simulink model "snap2_f_200msps_64i_4096c"  (R2019a)
settings: Solver=VariableStepDiscrete  StartTime=0.0  StopTime=10.0  RelTol=1e-3
undefined symbols (not defined in the file or in its folder): datetime, posixtime
libraries: xbsIndex_r4 x21354, casper_library_misc x297, casper_library_delays x19, xps_library x14, casper_library_sources x4
(part 17 of 217)

== system snap2_f_200msps_64i_4096c/cosmic_ray/count_thresh_exceeded2 ==
  pps_in : Inport
  din : Inport  Port=2
  AddSub : xbsIndex_r4/AddSub  mode=Subtraction  use_carryin=off  use_carryout=off  en=off  latency=1  precision=User Defined  arith_type=Unsigned  n_bits=5  bin_pt=0  quantization=Truncate  overflow=Wrap  use_behavioral_HDL=on  hw_selection=Fabric  pipelined=off  dbl_ovrd=off  block_type=addsub
  AddSub1 : xbsIndex_r4/AddSub  mode=Subtraction  use_carryin=off  use_carryout=off  en=off  latency=1  precision=User Defined  arith_type=Unsigned  n_bits=5  bin_pt=0  quantization=Truncate  overflow=Wrap  use_behavioral_HDL=on  hw_selection=Fabric  pipelined=off  dbl_ovrd=off  block_type=addsub
  Constant : xbsIndex_r4/Constant  const=32  gui_display_data_type=Fixed-point  arith_type=Unsigned  n_bits=6  bin_pt=0  preci_type=Single  exp_width=8  frac_width=24  explicit_period=off  period=1  equ=P=C  opselect=C  inp2=PCIN>>17  opr=+  inp1=P  carry=CIN  dbl_ovrd=off  block_type=constant
  Constant1 : xbsIndex_r4/Constant  const=1.0  gui_display_data_type=Fixed-point  arith_type=Unsigned  n_bits=1  bin_pt=0  preci_type=Single  exp_width=8  frac_width=24  explicit_period=off  period=1  equ=P=C  opselect=C  inp2=PCIN>>17  opr=+  inp1=P  carry=CIN  dbl_ovrd=off  block_type=constant
  Constant2 : xbsIndex_r4/Constant  const=1.0  gui_display_data_type=Fixed-point  arith_type=Unsigned  n_bits=1  bin_pt=0  preci_type=Single  exp_width=8  frac_width=24  explicit_period=off  period=1  equ=P=C  opselect=C  inp2=PCIN>>17  opr=+  inp1=P  carry=CIN  dbl_ovrd=off  block_type=constant
  Convert : xbsIndex_r4/Convert  gui_display_data_type=Boolean  arith_type=Boolean  n_bits=16  bin_pt=14  float_type=Single  exp_bits=8  fraction_bits=24  quantization=Truncate  overflow=Wrap  en=off  latency=1  pipeline=off  dbl_ovrd=off  block_type=convert
  Counter{2,6..68} (64 alike) : xbsIndex_r4/Counter  cnt_type=Count Limited  cnt_to=Inf  operation=Up  start_count=0  cnt_by_val=1  arith_type=Unsigned  n_bits=32  bin_pt=0  load_pin=off  rst=on  en=on  explicit_period=on  period=1  use_behavioral_HDL=off  implementation=Fabric  dbl_ovrd=off  block_type=counter
  Counter69 : xbsIndex_r4/Counter  cnt_type=Free Running  cnt_to=Inf  operation=Up  start_count=0  cnt_by_val=1  arith_type=Unsigned  n_bits=5  bin_pt=0  load_pin=off  rst=on  en=on  explicit_period=on  period=1  use_behavioral_HDL=off  implementation=Fabric  dbl_ovrd=off  block_type=counter
  Delay1 : xbsIndex_r4/Delay  rst=off  infoeditControl=Selection of Reset will increase slice count due to use of real FFs and instead of SRLs  en=off  latency=5  reg_retiming=on  dbl_ovrd=off  block_type=delay
  Delay10 : xbsIndex_r4/Delay  rst=off  infoeditControl=Selection of Reset will increase slice count due to use of real FFs and instead of SRLs  en=off  latency=13  reg_retiming=on  dbl_ovrd=off  block_type=delay
  Delay100 : xbsIndex_r4/Delay  rst=off  infoeditControl=Selection of Reset will increase slice count due to use of real FFs and instead of SRLs  en=off  latency=2  reg_retiming=on  dbl_ovrd=off  block_type=delay
  Delay101 : xbsIndex_r4/Delay  rst=off  infoeditControl=Selection of Reset will increase slice count due to use of real FFs and instead of SRLs  en=off  latency=3  reg_retiming=on  dbl_ovrd=off  block_type=delay
  Delay102 : xbsIndex_r4/Delay  rst=off  infoeditControl=Selection of Reset will increase slice count due to use of real FFs and instead of SRLs  en=off  latency=4  reg_retiming=on  dbl_ovrd=off  block_type=delay
  Delay11 : xbsIndex_r4/Delay  rst=off  infoeditControl=Selection of Reset will increase slice count due to use of real FFs and instead of SRLs  en=off  latency=14  reg_retiming=on  dbl_ovrd=off  block_type=delay
  Delay12 : xbsIndex_r4/Delay  rst=off  infoeditControl=Selection of Reset will increase slice count due to use of real FFs and instead of SRLs  en=off  latency=15  reg_retiming=on  dbl_ovrd=off  block_type=delay
  Delay13 : xbsIndex_r4/Delay  rst=off  infoeditControl=Selection of Reset will increase slice count due to use of real FFs and instead of SRLs  en=off  latency=16  reg_retiming=on  dbl_ovrd=off  block_type=delay
  Delay14 : xbsIndex_r4/Delay  rst=off  infoeditControl=Selection of Reset will increase slice count due to use of real FFs and instead of SRLs  en=off  latency=9  reg_retiming=on  dbl_ovrd=off  block_type=delay
  Delay15 : xbsIndex_r4/Delay  rst=off  infoeditControl=Selection of Reset will increase slice count due to use of real FFs and instead of SRLs  en=off  latency=10  reg_retiming=on  dbl_ovrd=off  block_type=delay
  Delay16 : xbsIndex_r4/Delay  rst=off  infoeditControl=Selection of Reset will increase slice count due to use of real FFs and instead of SRLs  en=off  latency=11  reg_retiming=on  dbl_ovrd=off  block_type=delay
  Delay17 : xbsIndex_r4/Delay  rst=off  infoeditControl=Selection of Reset will increase slice count due to use of real FFs and instead of SRLs  en=off  latency=12  reg_retiming=on  dbl_ovrd=off  block_type=delay
  Delay18 : xbsIndex_r4/Delay  rst=off  infoeditControl=Selection of Reset will increase slice count due to use of real FFs and instead of SRLs  en=off  latency=21  reg_retiming=on  dbl_ovrd=off  block_type=delay
  Delay19 : xbsIndex_r4/Delay  rst=off  infoeditControl=Selection of Reset will increase slice count due to use of real FFs and instead of SRLs  en=off  latency=22  reg_retiming=on  dbl_ovrd=off  block_type=delay
  Delay2 : xbsIndex_r4/Delay  rst=off  infoeditControl=Selection of Reset will increase slice count due to use of real FFs and instead of SRLs  en=off  latency=6  reg_retiming=on  dbl_ovrd=off  block_type=delay
  Delay20 : xbsIndex_r4/Delay  rst=off  infoeditControl=Selection of Reset will increase slice count due to use of real FFs and instead of SRLs  en=off  latency=23  reg_retiming=on  dbl_ovrd=off  block_type=delay
  Delay21 : xbsIndex_r4/Delay  rst=off  infoeditControl=Selection of Reset will increase slice count due to use of real FFs and instead of SRLs  en=off  latency=24  reg_retiming=on  dbl_ovrd=off  block_type=delay
  Delay22 : xbsIndex_r4/Delay  rst=off  infoeditControl=Selection of Reset will increase slice count due to use of real FFs and instead of SRLs  en=off  latency=29  reg_retiming=on  dbl_ovrd=off  block_type=delay
  Delay23 : xbsIndex_r4/Delay  rst=off  infoeditControl=Selection of Reset will increase slice count due to use of real FFs and instead of SRLs  en=off  latency=30  reg_retiming=on  dbl_ovrd=off  block_type=delay
  Delay24 : xbsIndex_r4/Delay  rst=off  infoeditControl=Selection of Reset will increase slice count due to use of real FFs and instead of SRLs  en=off  latency=31  reg_retiming=on  dbl_ovrd=off  block_type=delay
  Delay{25,34,38..40,70,99} (7 alike) : xbsIndex_r4/Delay  rst=off  infoeditControl=Selection of Reset will increase slice count due to use of real FFs and instead of SRLs  en=off  latency=1  reg_retiming=on  dbl_ovrd=off  block_type=delay
  Delay26 : xbsIndex_r4/Delay  rst=off  infoeditControl=Selection of Reset will increase slice count due to use of real FFs and instead of SRLs  en=off  latency=25  reg_retiming=on  dbl_ovrd=off  block_type=delay
  Delay27 : xbsIndex_r4/Delay  rst=off  infoeditControl=Selection of Reset will increase slice count due to use of real FFs and instead of SRLs  en=off  latency=26  reg_retiming=on  dbl_ovrd=off  block_type=delay
  Delay28 : xbsIndex_r4/Delay  rst=off  infoeditControl=Selection of Reset will increase slice count due to use of real FFs and instead of SRLs  en=off  latency=27  reg_retiming=on  dbl_ovrd=off  block_type=delay
  Delay29 : xbsIndex_r4/Delay  rst=off  infoeditControl=Selection of Reset will increase slice count due to use of real FFs and instead of SRLs  en=off  latency=28  reg_retiming=on  dbl_ovrd=off  block_type=delay
  Delay3 : xbsIndex_r4/Delay  rst=off  infoeditControl=Selection of Reset will increase slice count due to use of real FFs and instead of SRLs  en=off  latency=7  reg_retiming=on  dbl_ovrd=off  block_type=delay
  Delay30 : xbsIndex_r4/Delay  rst=off  infoeditControl=Selection of Reset will increase slice count due to use of real FFs and instead of SRLs  en=off  latency=17  reg_retiming=on  dbl_ovrd=off  block_type=delay
  Delay31 : xbsIndex_r4/Delay  rst=off  infoeditControl=Selection of Reset will increase slice count due to use of real FFs and instead of SRLs  en=off  latency=18  reg_retiming=on  dbl_ovrd=off  block_type=delay
  Delay32 : xbsIndex_r4/Delay  rst=off  infoeditControl=Selection of Reset will increase slice count due to use of real FFs and instead of SRLs  en=off  latency=19  reg_retiming=on  dbl_ovrd=off  block_type=delay
  Delay33 : xbsIndex_r4/Delay  rst=off  infoeditControl=Selection of Reset will increase slice count due to use of real FFs and instead of SRLs  en=off  latency=20  reg_retiming=on  dbl_ovrd=off  block_type=delay
  Delay35 : xbsIndex_r4/Delay  rst=off  infoeditControl=Selection of Reset will increase slice count due to use of real FFs and instead of SRLs  en=off  latency=2  reg_retiming=on  dbl_ovrd=off  block_type=delay
  Delay36 : xbsIndex_r4/Delay  rst=off  infoeditControl=Selection of Reset will increase slice count due to use of real FFs and instead of SRLs  en=off  latency=3  reg_retiming=on  dbl_ovrd=off  block_type=delay
  Delay37 : xbsIndex_r4/Delay  rst=off  infoeditControl=Selection of Reset will increase slice count due to use of real FFs and instead of SRLs  en=off  latency=4  reg_retiming=on  dbl_ovrd=off  block_type=delay
  Delay4 : xbsIndex_r4/Delay  rst=off  infoeditControl=Selection of Reset will increase slice count due to use of real FFs and instead of SRLs  en=off  latency=8  reg_retiming=on  dbl_ovrd=off  block_type=delay
  Delay5 : xbsIndex_r4/Delay  rst=off  infoeditControl=Selection of Reset will increase slice count due to use of real FFs and instead of SRLs  en=off  latency=13  reg_retiming=on  dbl_ovrd=off  block_type=delay
  Delay6 : xbsIndex_r4/Delay  rst=off  infoeditControl=Selection of Reset will increase slice count due to use of real FFs and instead of SRLs  en=off  latency=5  reg_retiming=on  dbl_ovrd=off  block_type=delay
  Delay7 : xbsIndex_r4/Delay  rst=off  infoeditControl=Selection of Reset will increase slice count due to use of real FFs and instead of SRLs  en=off  latency=6  reg_retiming=on  dbl_ovrd=off  block_type=delay
  Delay75 : xbsIndex_r4/Delay  rst=off  infoeditControl=Selection of Reset will increase slice count due to use of real FFs and instead of SRLs  en=off  latency=5  reg_retiming=on  dbl_ovrd=off  block_type=delay
  Delay76 : xbsIndex_r4/Delay  rst=off  infoeditControl=Selection of Reset will increase slice count due to use of real FFs and instead of SRLs  en=off  latency=14  reg_retiming=on  dbl_ovrd=off  block_type=delay
  Delay77 : xbsIndex_r4/Delay  rst=off  infoeditControl=Selection of Reset will increase slice count due to use of real FFs and instead of SRLs  en=off  latency=15  reg_retiming=on  dbl_ovrd=off  block_type=delay
  Delay78 : xbsIndex_r4/Delay  rst=off  infoeditControl=Selection of Reset will increase slice count due to use of real FFs and instead of SRLs  en=off  latency=16  reg_retiming=on  dbl_ovrd=off  block_type=delay
  Delay79 : xbsIndex_r4/Delay  rst=off  infoeditControl=Selection of Reset will increase slice count due to use of real FFs and instead of SRLs  en=off  latency=9  reg_retiming=on  dbl_ovrd=off  block_type=delay
  Delay8 : xbsIndex_r4/Delay  rst=off  infoeditControl=Selection of Reset will increase slice count due to use of real FFs and instead of SRLs  en=off  latency=7  reg_retiming=on  dbl_ovrd=off  block_type=delay
  Delay80 : xbsIndex_r4/Delay  rst=off  infoeditControl=Selection of Reset will increase slice count due to use of real FFs and instead of SRLs  en=off  latency=10  reg_retiming=on  dbl_ovrd=off  block_type=delay
  Delay81 : xbsIndex_r4/Delay  rst=off  infoeditControl=Selection of Reset will increase slice count due to use of real FFs and instead of SRLs  en=off  latency=11  reg_retiming=on  dbl_ovrd=off  block_type=delay
  Delay82 : xbsIndex_r4/Delay  rst=off  infoeditControl=Selection of Reset will increase slice count due to use of real FFs and instead of SRLs  en=off  latency=12  reg_retiming=on  dbl_ovrd=off  block_type=delay
  Delay83 : xbsIndex_r4/Delay  rst=off  infoeditControl=Selection of Reset will increase slice count due to use of real FFs and instead of SRLs  en=off  latency=21  reg_retiming=on  dbl_ovrd=off  block_type=delay
  Delay84 : xbsIndex_r4/Delay  rst=off  infoeditControl=Selection of Reset will increase slice count due to use of real FFs and instead of SRLs  en=off  latency=22  reg_retiming=on  dbl_ovrd=off  block_type=delay
  Delay85 : xbsIndex_r4/Delay  rst=off  infoeditControl=Selection of Reset will increase slice count due to use of real FFs and instead of SRLs  en=off  latency=23  reg_retiming=on  dbl_ovrd=off  block_type=delay
  Delay86 : xbsIndex_r4/Delay  rst=off  infoeditControl=Selection of Reset will increase slice count due to use of real FFs and instead of SRLs  en=off  latency=24  reg_retiming=on  dbl_ovrd=off  block_type=delay
  Delay87 : xbsIndex_r4/Delay  rst=off  infoeditControl=Selection of Reset will increase slice count due to use of real FFs and instead of SRLs  en=off  latency=29  reg_retiming=on  dbl_ovrd=off  block_type=delay
  Delay88 : xbsIndex_r4/Delay  rst=off  infoeditControl=Selection of Reset will increase slice count due to use of real FFs and instead of SRLs  en=off  latency=30  reg_retiming=on  dbl_ovrd=off  block_type=delay
  Delay89 : xbsIndex_r4/Delay  rst=off  infoeditControl=Selection of Reset will increase slice count due to use of real FFs and instead of SRLs  en=off  latency=31  reg_retiming=on  dbl_ovrd=off  block_type=delay
  Delay9 : xbsIndex_r4/Delay  rst=off  infoeditControl=Selection of Reset will increase slice count due to use of real FFs and instead of SRLs  en=off  latency=8  reg_retiming=on  dbl_ovrd=off  block_type=delay
  Delay91 : xbsIndex_r4/Delay  rst=off  infoeditControl=Selection of Reset will increase slice count due to use of real FFs and instead of SRLs  en=off  latency=25  reg_retiming=on  dbl_ovrd=off  block_type=delay
  Delay92 : xbsIndex_r4/Delay  rst=off  infoeditControl=Selection of Reset will increase slice count due to use of real FFs and instead of SRLs  en=off  latency=26  reg_retiming=on  dbl_ovrd=off  block_type=delay
  Delay93 : xbsIndex_r4/Delay  rst=off  infoeditControl=Selection of Reset will increase slice count due to use of real FFs and instead of SRLs  en=off  latency=27  reg_retiming=on  dbl_ovrd=off  block_type=delay
  Delay94 : xbsIndex_r4/Delay  rst=off  infoeditControl=Selection of Reset will increase slice count due to use of real FFs and instead of SRLs  en=off  latency=28  reg_retiming=on  dbl_ovrd=off  block_type=delay
  Delay95 : xbsIndex_r4/Delay  rst=off  infoeditControl=Selection of Reset will increase slice count due to use of real FFs and instead of SRLs  en=off  latency=17  reg_retiming=on  dbl_ovrd=off  block_type=delay
  Delay96 : xbsIndex_r4/Delay  rst=off  infoeditControl=Selection of Reset will increase slice count due to use of real FFs and instead of SRLs  en=off  latency=18  reg_retiming=on  dbl_ovrd=off  block_type=delay
  Delay97 : xbsIndex_r4/Delay  rst=off  infoeditControl=Selection of Reset will increase slice count due to use of real FFs and instead of SRLs  en=off  latency=19  reg_retiming=on  dbl_ovrd=off  block_type=delay
  Delay98 : xbsIndex_r4/Delay  rst=off  infoeditControl=Selection of Reset will increase slice count due to use of real FFs and instead of SRLs  en=off  latency=20  reg_retiming=on  dbl_ovrd=off  block_type=delay
  Mux : xbsIndex_r4/Mux  inputs=32  en=off  latency=1  precision=Full  arith_type=Unsigned  n_bits=16  bin_pt=14  quantization=Truncate  overflow=Wrap  dbl_ovrd=off  block_type=mux
  Mux1 : xbsIndex_r4/Mux  inputs=32  en=off  latency=1  precision=Full  arith_type=Unsigned  n_bits=16  bin_pt=14  quantization=Truncate  overflow=Wrap  dbl_ovrd=off  block_type=mux
  bus_expand : Subsystem  AncestorBlock=casper_library_flow_control/bus_expand  mask(bus_expand){mode=divisions of equal size, outputNum=64, outputWidth=1, outputBinaryPt=0, outputArithmeticType=2, show_format=off, outputToWorkspace=off, variablePrefix=out, outputToModelAsWell=on}
      mask prompts: outputNum "Number of outputs:"; outputWidth "Output width:"; outputBinaryPt "Output binary point position:"; outputArithmeticType "Output arithmetic type (ufix=0, fix=1, bool=2):"; show_format "Print format string?"; outputToWorkspace "Output to workspace?"; variablePrefix "Variable name prefix:"; outputToModelAsWell "Output to model as well?"
      mask help:
      | Expands a 'bus' made using a bus_create or Xilinx
      | concat block.
      | The input will be divided into the specified number
      | of outputs with the specified arithmetic types.
      | Divisions are made from most significant bit.
      mask init: same as snap2_f_200msps_64i_4096c/autocorr/bus_expand
      settings: AttributesFormatString=64 outputs
      mask TypeOptions mode: divisions of equal size | divisions of arbitrary size
      mask Callback mode: bus_expand_callback();
      mask Callback outputWidth: bus_expand_callback();
      mask Callback outputToWorkspace: bus_expand_callback();
  custom_pulse_extend1 : Subsystem
  edge_detect : casper_library_misc/edge_detect  edge=Rising  polarity=Active High  x_in=[0 0.08 0.08 0.16 0.16 0.24 0.24 0.32 0.32 0.4]  y_in="[-1 -1  1  1  1  1  1  1  1  1]"  x_out=[0.6 0.68 0.68 0.76 0.76 0.84 0.84 0.92 0.92 1]  y_out="[-1 -1  1  1 -1 -1 -1 -1 -1 -1]"
  addr1 : Outport
  dout1 : Outport  Port=2
  we1 : Outport  Port=3
  addr2 : Outport  Port=4
  dout2 : Outport  Port=5
  we2 : Outport  Port=6
  wires:
  Mux1/1 -> Delay39/1
  [count_bram_we] -> Delay40/1
  Delay39/1 -> dout2/1
  Delay40/1 -> we2/1
  Constant2/1 -> AddSub1/2
  AddSub1/1 -> addr2/1
  [count_bram_addr] -> AddSub1/1
  [count_bram_addr] -> AddSub/1
  AddSub/1 -> addr1/1
  Constant1/1 -> AddSub/2
  Delay38/1 -> we1/1
  Delay25/1 -> dout1/1
  Mux/1 -> Delay25/1
  [count_bram_we] -> Delay38/1
  Counter65/1 -> Delay34/1
  Delay23/1 -> Mux1/32
  Delay76/1 -> Mux/16
  Counter55/1 -> Delay21/1
  Counter15/1 -> Delay77/1
  bus_expand/6(out59) -> Counter10/2
  Counter43/1 -> Delay9/1
  Counter41/1 -> Delay11/1
  Delay18/1 -> Mux1/23
  bus_expand/4(out61) -> Counter8/2
  Counter38/1 -> Delay7/1
  Delay1/1 -> Mux/7
  Delay34/1 -> Mux1/3
  Counter25/1 -> Delay88/1
  Counter16/1 -> Delay4/1
  Delay24/1 -> Mux1/33
  Delay88/1 -> Mux/32
  Delay80/1 -> Mux/12
  Counter34/1 -> Delay96/1
  Delay2/1 -> Mux/8
  bus_expand/30(out35) -> Counter24/2
  bus_expand/16(out49) -> Counter15/2
  Counter58/1 -> Delay28/1
  Delay81/1 -> Mux/13
  Counter13/1 -> Delay5/1
  Delay32/1 -> Mux1/21
  Counter42/1 -> Delay12/1
  bus_expand/49(out16) -> Counter59/2
  bus_expand/54(out11) -> Counter49/2
  Delay75/1 -> Counter2/1, Counter6/1, Counter7/1, Counter8/1, Counter9/1, Counter10/1, Counter11/1, Counter12/1, Counter16/1, Counter15/1, Counter31/1, Counter28/1, Counter29/1, Counter30/1, Counter32/1, Counter24/1, Counter25/1, Counter26/1, Counter44/1, Counter45/1, Counter46/1, Counter48/1, Counter40/1, Counter41/1, Counter61/1, Counter62/1, Counter63/1, Counter64/1, Counter49/1, Counter50/1, Counter51/1, Counter55/1, Counter54/1, Counter53/1, Counter52/1, Counter60/1, Counter58/1, Counter57/1, Counter56/1, Counter59/1, Counter42/1, Counter43/1, Counter39/1, Counter38/1, Counter37/1, Counter68/1, Counter67/1, Counter66/1, Counter65/1, Counter47/1, Counter27/1, Counter23/1, Counter22/1, Counter21/1, Counter36/1, Counter35/1, Counter34/1, Counter33/1, Counter14/1, Counter13/1, Counter20/1, Counter19/1, Counter18/1, Counter17/1
  Counter40/1 -> Delay10/1
  bus_expand/22(out43) -> Counter21/2
  Counter56/1 -> Delay26/1
  bus_expand/58(out7) -> Counter56/2
  Delay78/1 -> Mux/18
  bus_expand/34(out31) -> Counter65/2
  Delay100/1 -> Mux/4
  Counter8/1 -> Delay101/1
  Delay6/1 -> Mux1/7
  Delay85/1 -> Mux/25
  Counter66/1 -> Delay35/1
  Delay27/1 -> Mux1/28
  Counter21/1 -> Delay83/1
  Counter17/1 -> Delay79/1
  Counter63/1 -> Delay32/1
  Delay93/1 -> Mux/29
  Counter48/1 -> Delay17/1
  bus_expand/35(out30) -> Counter66/2
  bus_expand/61(out4) -> Counter60/2
  Delay99/1 -> Mux/3
  bus_expand/9(out56) -> Counter16/2
  bus_expand/28(out37) -> Counter30/2
  Delay21/1 -> Mux1/26
  Counter59/1 -> Delay13/1
  Counter14/1 -> Delay76/1
  bus_expand/40(out25) -> Counter39/2
  Delay12/1 -> Mux1/17
  Delay7/1 -> Mux1/8
  Delay4/1 -> Mux/10
  bus_expand/18(out47) -> Counter33/2
  Delay17/1 -> Mux1/14
  Counter30/1 -> Delay93/1
  Delay3/1 -> Mux/9
  Counter53/1 -> Delay23/1
  Delay37/1 -> Mux1/6
  Counter24/1 -> Delay87/1
  Counter45/1 -> Delay15/1
  Counter7/1 -> Delay100/1
  Delay92/1 -> Mux/28
  bus_expand/57(out8) -> Counter55/2
  Counter51/1 -> Delay20/1
  Delay98/1 -> Mux/22
  Counter64/1 -> Delay33/1
  Counter52/1 -> Delay22/1
  Counter67/1 -> Delay36/1
  Delay14/1 -> Mux1/11
  bus_expand/52(out13) -> Counter63/2
  Counter37/1 -> Delay6/1
  Counter60/1 -> Delay29/1
  bus_expand/14(out51) -> Counter13/2
  Delay22/1 -> Mux1/31
  Counter35/1 -> Delay97/1
  bus_expand/59(out6) -> Counter57/2
  bus_expand/43(out22) -> Counter45/2
  Delay91/1 -> Mux/27
  Counter36/1 -> Delay98/1
  Counter23/1 -> Delay85/1
  Counter47/1 -> Mux1/2
  Counter26/1 -> Delay89/1
  bus_expand/15(out50) -> Counter14/2
  bus_expand/7(out58) -> Counter11/2
  Delay35/1 -> Mux1/4
  Counter18/1 -> Delay80/1
  bus_expand/36(out29) -> Counter67/2
  bus_expand/46(out19) -> Counter40/2
  Counter49/1 -> Delay18/1
  bus_expand/55(out10) -> Counter50/2
  Delay86/1 -> Mux/26
  bus_expand/44(out21) -> Counter46/2
  Delay26/1 -> Mux1/27
  Counter11/1 -> Delay2/1
  Delay16/1 -> Mux1/13
  bus_expand/23(out42) -> Counter22/2
  Delay20/1 -> Mux1/25
  bus_expand/21(out44) -> Counter36/2
  din/1 -> bus_expand/1(bus_in)
  Delay13/1 -> Mux1/18
  Counter50/1 -> Delay19/1
  Delay10/1 -> Mux1/15
  bus_expand/2(out63) -> Counter6/2
  Delay79/1 -> Mux/11
  bus_expand/3(out62) -> Counter7/2
  Counter27/1 -> Delay86/1
  Delay30/1 -> Mux1/19
  bus_expand/48(out17) -> Counter42/2
  Counter61/1 -> Delay30/1
  Counter22/1 -> Delay84/1
  Counter12/1 -> Delay3/1
  bus_expand/41(out24) -> Counter43/2
  bus_expand/39(out26) -> Counter38/2
  Counter10/1 -> Delay1/1
  bus_expand/31(out34) -> Counter25/2
  Delay89/1 -> Mux/33
  bus_expand/12(out53) -> Counter19/2
  bus_expand/51(out14) -> Counter62/2
  Delay84/1 -> Mux/24
  Counter19/1 -> Delay81/1
  Delay95/1 -> Mux/19
  Delay19/1 -> Mux1/24
  bus_expand/62(out3) -> Counter52/2
  bus_expand/63(out2) -> Counter53/2
  Delay8/1 -> Mux1/9
  Counter32/1 -> Delay94/1
  Delay96/1 -> Mux/20
  Counter28/1 -> Delay91/1
  bus_expand/10(out55) -> Counter17/2
  Counter33/1 -> Delay95/1
  Counter9/1 -> Delay102/1
  Delay97/1 -> Mux/21
  bus_expand/8(out57) -> Counter12/2
  Delay11/1 -> Mux1/16
  Counter57/1 -> Delay27/1
  Counter44/1 -> Delay14/1
  Delay5/1 -> Mux/15
  Delay102/1 -> Mux/6
  bus_expand/37(out28) -> Counter68/2
  Delay29/1 -> Mux1/30
  bus_expand/60(out5) -> Counter58/2
  Counter31/1 -> Delay78/1
  bus_expand/45(out20) -> Counter48/2
  Delay82/1 -> Mux/14
  bus_expand/47(out18) -> Counter41/2
  Counter20/1 -> Delay82/1
  Counter46/1 -> Delay16/1
  bus_expand/38(out27) -> Counter37/2
  Counter62/1 -> Delay31/1
  bus_expand/29(out36) -> Counter32/2
  bus_expand/33(out32) -> Counter47/2
  Counter68/1 -> Delay37/1
  Delay87/1 -> Mux/31
  bus_expand/25(out40) -> Counter27/2
  bus_expand/17(out48) -> Counter31/2
  bus_expand/26(out39) -> Counter28/2
  bus_expand/56(out9) -> Counter51/2
  Counter39/1 -> Delay8/1
  bus_expand/13(out52) -> Counter20/2
  Delay77/1 -> Mux/17
  Delay33/1 -> Mux1/22
  Delay31/1 -> Mux1/20
  bus_expand/11(out54) -> Counter18/2
  Delay28/1 -> Mux1/29
  bus_expand/32(out33) -> Counter26/2
  Counter29/1 -> Delay92/1
  bus_expand/53(out12) -> Counter64/2
  Delay83/1 -> Mux/23
  bus_expand/24(out41) -> Counter23/2
  Delay101/1 -> Mux/5
  bus_expand/27(out38) -> Counter29/2
  [count_bram_addr] -> Mux1/1
  bus_expand/42(out23) -> Counter44/2
  Delay70/1 -> [count_bram_we]
  bus_expand/19(out46) -> Counter34/2
  Delay9/1 -> Mux1/10
  Delay36/1 -> Mux1/5
  bus_expand/5(out60) -> Counter9/2
  bus_expand/50(out15) -> Counter61/2
  Counter6/1 -> Delay99/1
  Delay15/1 -> Mux1/12
  bus_expand/20(out45) -> Counter35/2
  Delay94/1 -> Mux/30
  Counter54/1 -> Delay24/1
  bus_expand/64(lsb_out1) -> Counter54/2
  bus_expand/1(msb_out64) -> Counter2/2
  Counter2/1 -> Mux/2
  [count_bram_addr] -> Mux/1
  custom_pulse_extend1/1("out ") -> Convert/1
  Constant/1 -> custom_pulse_extend1/2("pulse_length ")
  Counter69/1 -> [count_bram_addr]
  Convert/1 -> Delay70/1, Counter69/2
  pps_in/1 -> edge_detect/1
  edge_detect/1 -> Counter69/1, Delay75/1, custom_pulse_extend1/1("in ")

== system snap2_f_200msps_64i_4096c/cosmic_ray/count_triggers ==
  pps : Inport
  din1 : Inport  Port=2
  din2 : Inport  Port=3
  Constant : xbsIndex_r4/Constant  const=2  gui_display_data_type=Fixed-point  arith_type=Unsigned  n_bits=2  bin_pt=0  preci_type=Single  exp_width=8  frac_width=24  explicit_period=off  period=1  equ=P=C  opselect=C  inp2=PCIN>>17  opr=+  inp1=P  carry=CIN  dbl_ovrd=off  block_type=constant
  Convert : xbsIndex_r4/Convert  gui_display_data_type=Boolean  arith_type=Boolean  n_bits=16  bin_pt=14  float_type=Single  exp_bits=8  fraction_bits=24  quantization=Truncate  overflow=Wrap  en=off  latency=1  pipeline=off  dbl_ovrd=off  block_type=convert
  Counter2 : xbsIndex_r4/Counter  cnt_type=Count Limited  cnt_to=Inf  operation=Up  start_count=0  cnt_by_val=1  arith_type=Unsigned  n_bits=32  bin_pt=0  load_pin=off  rst=on  en=on  explicit_period=on  period=1  use_behavioral_HDL=off  implementation=Fabric  dbl_ovrd=off  block_type=counter
  Counter6 : xbsIndex_r4/Counter  cnt_type=Count Limited  cnt_to=Inf  operation=Up  start_count=0  cnt_by_val=1  arith_type=Unsigned  n_bits=32  bin_pt=0  load_pin=off  rst=on  en=on  explicit_period=on  period=1  use_behavioral_HDL=off  implementation=Fabric  dbl_ovrd=off  block_type=counter
  Counter69 : xbsIndex_r4/Counter  cnt_type=Free Running  cnt_to=Inf  operation=Up  start_count=0  cnt_by_val=1  arith_type=Unsigned  n_bits=1  bin_pt=0  load_pin=off  rst=on  en=on  explicit_period=on  period=1  use_behavioral_HDL=off  implementation=Fabric  dbl_ovrd=off  block_type=counter
  Delay70 : xbsIndex_r4/Delay  rst=off  infoeditControl=Selection of Reset will increase slice count due to use of real FFs and instead of SRLs  en=off  latency=1  reg_retiming=on  dbl_ovrd=off  block_type=delay
  Delay75 : xbsIndex_r4/Delay  rst=off  infoeditControl=Selection of Reset will increase slice count due to use of real FFs and instead of SRLs  en=off  latency=5  reg_retiming=on  dbl_ovrd=off  block_type=delay
  Delay99 : xbsIndex_r4/Delay  rst=off  infoeditControl=Selection of Reset will increase slice count due to use of real FFs and instead of SRLs  en=off  latency=1  reg_retiming=on  dbl_ovrd=off  block_type=delay
  Mux : xbsIndex_r4/Mux  inputs=2  en=off  latency=1  precision=Full  arith_type=Unsigned  n_bits=16  bin_pt=14  quantization=Truncate  overflow=Wrap  dbl_ovrd=off  block_type=mux
  Scope : Scope  Commented=on
  Scope1 : Scope  Commented=on
  custom_pulse_extend1 : Subsystem
  edge_detect : casper_library_misc/edge_detect  edge=Rising  polarity=Active High  x_in=[0 0.08 0.08 0.16 0.16 0.24 0.24 0.32 0.32 0.4]  y_in="[-1 -1  1  1  1  1  1  1  1  1]"  x_out=[0.6 0.68 0.68 0.76 0.76 0.84 0.84 0.92 0.92 1]  y_out="[-1 -1  1  1 -1 -1 -1 -1 -1 -1]"
  "addr " : Outport
  dout : Outport  Port=2
  "we " : Outport  Port=3
  wires:
  din2/1 -> Counter6/2
  edge_detect/1 -> custom_pulse_extend1/1("in "), Delay75/1, Counter69/1
  Constant/1 -> custom_pulse_extend1/2("pulse_length ")
  [count_bram_addr] -> Mux/1
  Counter2/1 -> Scope1/1, Mux/2
  Convert/1 -> Counter69/2, Delay70/1
  Delay70/1 -> [count_bram_we]
  [count_bram_we] -> "we "/1
  Counter6/1 -> Delay99/1
  din1/1 -> Counter2/2
  pps/1 -> edge_detect/1
  Delay99/1 -> Scope/1, Mux/3
  Delay75/1 -> Counter6/1, Counter2/1
  custom_pulse_extend1/1("out ") -> Convert/1
  Counter69/1 -> [count_bram_addr]
  Mux/1 -> dout/1
  [count_bram_addr] -> "addr "/1

== system snap2_f_200msps_64i_4096c/cosmic_ray/counter_test_signal1 ==
  bus_create : Subsystem  AncestorBlock=casper_library_flow_control/bus_create  mask(bus_create){inputNum=16}
      mask prompts: inputNum "Number of inputs:"
      mask init:
      | bus_create_init(gcb,...
      |     'inputNum', inputNum);
  bus_create1 : Subsystem  AncestorBlock=casper_library_flow_control/bus_create  mask(bus_create){inputNum=16}
      mask prompts: inputNum "Number of inputs:"
      mask init:
      | bus_create_init(gcb,...
      |     'inputNum', inputNum);
  bus_create2 : Subsystem  AncestorBlock=casper_library_flow_control/bus_create  mask(bus_create){inputNum=16}
      mask prompts: inputNum "Number of inputs:"
      mask init:
      | bus_create_init(gcb,...
      |     'inputNum', inputNum);
  bus_create3 : Subsystem  AncestorBlock=casper_library_flow_control/bus_create  mask(bus_create){inputNum=16}
      mask prompts: inputNum "Number of inputs:"
      mask init:
      | bus_create_init(gcb,...
      |     'inputNum', inputNum);
  bus_create4 : Subsystem  AncestorBlock=casper_library_flow_control/bus_create  mask(bus_create){inputNum=4}
      mask prompts: inputNum "Number of inputs:"
      mask init:
      | bus_create_init(gcb,...
      |     'inputNum', inputNum);
  testvec1 : xbsIndex_r4/Counter  cnt_type=Free Running  cnt_to=Inf  operation=Up  start_count=0  cnt_by_val=1  arith_type="Signed  (2's comp)"  n_bits=10  bin_pt=0  load_pin=off  rst=off  en=off  explicit_period=on  period=1  use_behavioral_HDL=off  implementation=Fabric  dbl_ovrd=off  block_type=counter
  Out1 : Outport
  wires:
  bus_create4/1(bus_out) -> Out1/1
  bus_create3/1(bus_out) -> bus_create4/4(in4)
  bus_create2/1(bus_out) -> bus_create4/2(in2)
  bus_create/1(bus_out) -> bus_create4/1(in1)
  testvec1/1 -> bus_create/16(in16), bus_create/15(in15), bus_create/14(in14), bus_create/13(in13), bus_create/12(in12), bus_create/11(in11), bus_create/10(in10), bus_create/9(in9), bus_create/8(in8), bus_create/7(in7), bus_create/6(in6), bus_create/5(in5), bus_create/4(in4), bus_create/3(in3), bus_create/2(in2), bus_create/1(in1), bus_create3/1(in1), bus_create3/2(in2), bus_create3/3(in3), bus_create3/5(in5), bus_create3/6(in6), bus_create3/7(in7), bus_create3/8(in8), bus_create3/9(in9), bus_create3/11(in11), bus_create3/12(in12), bus_create3/13(in13), bus_create3/15(in15), bus_create3/16(in16), bus_create3/14(in14), bus_create3/10(in10), bus_create3/4(in4), bus_create1/16(in16), bus_create1/1(in1), bus_create1/15(in15), bus_create1/14(in14), bus_create1/2(in2), bus_create1/13(in13), bus_create1/3(in3), bus_create1/4(in4), bus_create1/12(in12), bus_create1/11(in11), bus_create1/5(in5), bus_create1/10(in10), bus_create1/6(in6), bus_create1/9(in9), bus_create1/7(in7), bus_create1/8(in8), bus_create2/16(in16), bus_create2/15(in15), bus_create2/14(in14), bus_create2/13(in13), bus_create2/12(in12), bus_create2/11(in11), bus_create2/10(in10), bus_create2/9(in9), bus_create2/7(in7), bus_create2/6(in6), bus_create2/5(in5), bus_create2/4(in4), bus_create2/3(in3), bus_create2/2(in2), bus_create2/1(in1), bus_create2/8(in8)
  bus_create1/1(bus_out) -> bus_create4/3(in3)

== system snap2_f_200msps_64i_4096c/cosmic_ray/cr_coinc_thresh ==
  sim_1 : Inport
  convert1_1 : DataTypeConversion  OutDataTypeStr=fixdt('ufix32_En0')  LockScale=on
  convert2_1 : DataTypeConversion  OutDataTypeStr=fixdt('ufix32_En0')  ConvertRealWorld=Stored Integer (SI)  LockScale=on
  gain_1 : Gain
  io_delay : xbsIndex_r4/Delay  rst=off  infoeditControl=Selection of Reset will increase slice count due to use of real FFs and instead of SRLs  en=off  latency=0  reg_retiming=on  dbl_ovrd=off  block_type=delay
  reint1 : xbsIndex_r4/Reinterpret  force_arith_type=on  arith_type=Unsigned  force_bin_pt=on  bin_pt=0  block_type=reinterpret
  slice_reg : xbsIndex_r4/Slice  nbits=32  boolean_output=off  mode=Lower Bit Location + Width  bit1=0  base1=MSB of Input  bit0=0  base0=LSB of Input  dbl_ovrd=off  block_type=slice
  snap2_f_200msps_64i_4096c_cosmic_ray_cr_coinc_thresh_user_data_out : xbsIndex_r4/Gateway In  gui_display_data_type=Fixed-point  arith_type=Unsigned  n_bits=32  bin_pt=0  preci_type=Single  exp_width=8  frac_width=24  rows=1  columns=1  quantization="Round  (unbiased: +/- Inf)"  overflow=Saturate  period=1  UseAsADC=off  ADCChannel='1'  interface=None  automatic_assignment=on  address_offset=hex2dec('00')  intf_name=''  intf_description=''  default_value=0  timing_constraint=None  locs_specified=off  LOCs={}  io_standard={}  inherit_from_input=off  hdl_port=on  dbl_ovrd=off  block_type=gatewayin
  in_reg : Outport
  wires:
  snap2_f_200msps_64i_4096c_cosmic_ray_cr_coinc_thresh_user_data_out/1 -> io_delay/1
  sim_1/1 -> convert1_1/1
  convert1_1/1 -> convert2_1/1
  convert2_1/1 -> gain_1/1
  gain_1/1 -> snap2_f_200msps_64i_4096c_cosmic_ray_cr_coinc_thresh_user_data_out/1
  io_delay/1 -> slice_reg/1
  slice_reg/1 -> reint1/1
  reint1/1 -> in_reg/1

== system snap2_f_200msps_64i_4096c/cosmic_ray/cr_coinc_window ==
  sim_1 : Inport
  convert1_1 : DataTypeConversion  OutDataTypeStr=fixdt('ufix32_En0')  LockScale=on
  convert2_1 : DataTypeConversion  OutDataTypeStr=fixdt('ufix32_En0')  ConvertRealWorld=Stored Integer (SI)  LockScale=on
  gain_1 : Gain
  io_delay : xbsIndex_r4/Delay  rst=off  infoeditControl=Selection of Reset will increase slice count due to use of real FFs and instead of SRLs  en=off  latency=0  reg_retiming=on  dbl_ovrd=off  block_type=delay
  reint1 : xbsIndex_r4/Reinterpret  force_arith_type=on  arith_type=Unsigned  force_bin_pt=on  bin_pt=0  block_type=reinterpret
  slice_reg : xbsIndex_r4/Slice  nbits=32  boolean_output=off  mode=Lower Bit Location + Width  bit1=0  base1=MSB of Input  bit0=0  base0=LSB of Input  dbl_ovrd=off  block_type=slice
  snap2_f_200msps_64i_4096c_cosmic_ray_cr_coinc_window_user_data_out : xbsIndex_r4/Gateway In  gui_display_data_type=Fixed-point  arith_type=Unsigned  n_bits=32  bin_pt=0  preci_type=Single  exp_width=8  frac_width=24  rows=1  columns=1  quantization="Round  (unbiased: +/- Inf)"  overflow=Saturate  period=1  UseAsADC=off  ADCChannel='1'  interface=None  automatic_assignment=on  address_offset=hex2dec('00')  intf_name=''  intf_description=''  default_value=0  timing_constraint=None  locs_specified=off  LOCs={}  io_standard={}  inherit_from_input=off  hdl_port=on  dbl_ovrd=off  block_type=gatewayin
  in_reg : Outport
  wires:
  snap2_f_200msps_64i_4096c_cosmic_ray_cr_coinc_window_user_data_out/1 -> io_delay/1
  sim_1/1 -> convert1_1/1
  convert1_1/1 -> convert2_1/1
  convert2_1/1 -> gain_1/1
  gain_1/1 -> snap2_f_200msps_64i_4096c_cosmic_ray_cr_coinc_window_user_data_out/1
  io_delay/1 -> slice_reg/1
  slice_reg/1 -> reint1/1
  reint1/1 -> in_reg/1

== system snap2_f_200msps_64i_4096c/cosmic_ray/cr_dest_ip ==
  sim_1 : Inport
  convert1_1 : DataTypeConversion  OutDataTypeStr=fixdt('ufix32_En0')  LockScale=on
  convert2_1 : DataTypeConversion  OutDataTypeStr=fixdt('ufix32_En0')  ConvertRealWorld=Stored Integer (SI)  LockScale=on
  gain_1 : Gain
  io_delay : xbsIndex_r4/Delay  rst=off  infoeditControl=Selection of Reset will increase slice count due to use of real FFs and instead of SRLs  en=off  latency=0  reg_retiming=on  dbl_ovrd=off  block_type=delay
  reint1 : xbsIndex_r4/Reinterpret  force_arith_type=on  arith_type=Unsigned  force_bin_pt=on  bin_pt=0  block_type=reinterpret
  slice_reg : xbsIndex_r4/Slice  nbits=32  boolean_output=off  mode=Lower Bit Location + Width  bit1=0  base1=MSB of Input  bit0=0  base0=LSB of Input  dbl_ovrd=off  block_type=slice
  snap2_f_200msps_64i_4096c_cosmic_ray_cr_dest_ip_user_data_out : xbsIndex_r4/Gateway In  gui_display_data_type=Fixed-point  arith_type=Unsigned  n_bits=32  bin_pt=0  preci_type=Single  exp_width=8  frac_width=24  rows=1  columns=1  quantization="Round  (unbiased: +/- Inf)"  overflow=Saturate  period=1  UseAsADC=off  ADCChannel='1'  interface=None  automatic_assignment=on  address_offset=hex2dec('00')  intf_name=''  intf_description=''  default_value=0  timing_constraint=None  locs_specified=off  LOCs={}  io_standard={}  inherit_from_input=off  hdl_port=on  dbl_ovrd=off  block_type=gatewayin
  in_reg : Outport
  wires:
  snap2_f_200msps_64i_4096c_cosmic_ray_cr_dest_ip_user_data_out/1 -> io_delay/1
  sim_1/1 -> convert1_1/1
  convert1_1/1 -> convert2_1/1
  convert2_1/1 -> gain_1/1
  gain_1/1 -> snap2_f_200msps_64i_4096c_cosmic_ray_cr_dest_ip_user_data_out/1
  io_delay/1 -> slice_reg/1
  slice_reg/1 -> reint1/1
  reint1/1 -> in_reg/1

== system snap2_f_200msps_64i_4096c/cosmic_ray/cr_dest_port ==
  sim_1 : Inport
  convert1_1 : DataTypeConversion  OutDataTypeStr=fixdt('ufix16_En0')  LockScale=on
  convert2_1 : DataTypeConversion  OutDataTypeStr=fixdt('ufix16_En0')  ConvertRealWorld=Stored Integer (SI)  LockScale=on
  gain_1 : Gain
  io_delay : xbsIndex_r4/Delay  rst=off  infoeditControl=Selection of Reset will increase slice count due to use of real FFs and instead of SRLs  en=off  latency=0  reg_retiming=on  dbl_ovrd=off  block_type=delay
  reint1 : xbsIndex_r4/Reinterpret  force_arith_type=on  arith_type=Unsigned  force_bin_pt=on  bin_pt=0  block_type=reinterpret
  slice_reg : xbsIndex_r4/Slice  nbits=16  boolean_output=off  mode=Lower Bit Location + Width  bit1=0  base1=MSB of Input  bit0=0  base0=LSB of Input  dbl_ovrd=off  block_type=slice
  snap2_f_200msps_64i_4096c_cosmic_ray_cr_dest_port_user_data_out : xbsIndex_r4/Gateway In  gui_display_data_type=Fixed-point  arith_type=Unsigned  n_bits=32  bin_pt=0  preci_type=Single  exp_width=8  frac_width=24  rows=1  columns=1  quantization="Round  (unbiased: +/- Inf)"  overflow=Saturate  period=1  UseAsADC=off  ADCChannel='1'  interface=None  automatic_assignment=on  address_offset=hex2dec('00')  intf_name=''  intf_description=''  default_value=0  timing_constraint=None  locs_specified=off  LOCs={}  io_standard={}  inherit_from_input=off  hdl_port=on  dbl_ovrd=off  block_type=gatewayin
  in_reg : Outport
  wires:
  snap2_f_200msps_64i_4096c_cosmic_ray_cr_dest_port_user_data_out/1 -> io_delay/1
  sim_1/1 -> convert1_1/1
  convert1_1/1 -> convert2_1/1
  convert2_1/1 -> gain_1/1
  gain_1/1 -> snap2_f_200msps_64i_4096c_cosmic_ray_cr_dest_port_user_data_out/1
  io_delay/1 -> slice_reg/1
  slice_reg/1 -> reint1/1
  reint1/1 -> in_reg/1
